simulink model "cSPACE_28335demo"  (R2017a)
settings: Solver=FixedStepDiscrete  StartTime=0.0  StopTime=inf  FixedStep=0.005  RelTol=1e-3  EnableMultiTasking=on
PostLoadFcn:
  | c2000demoscallback(1)
undefined symbols (not defined in the file or in its folder): Hardware_Interface, WM_DA0
libraries: idelinklib_common x16, simulink x4, c280xlib x2, c2833xlib x1
settings Model: ExtModeTrigDuration=8  Creator=The MathWorks Inc.  LastModifiedBy=307
settings DataIOCC: LimitDataPoints=on  SaveFormat=Array  SignalLoggingSaveFormat=ModelDataLogs  SaveOutput=off  SaveTime=off  SignalLoggingName=sigsOut
settings OptimizationCC: DefaultUnderspecifiedDataType=single  ExpressionDepthLimit=2147483647  InitFltsAndDblsToZero=on  LifeSpan=inf  MaxStackSize=512
settings DebuggingCC: UnderspecifiedInitializationDetection=Classic  MergeDetectMultiDrivingBlocksExec=none  CheckExecutionContextPreStartOutputMsg=on  CheckExecutionContextRuntimeOutputMsg=on  SignalResolutionControl=TryResolveAllWithWarning  MultiTaskDSMMsg=warning  MultiTaskCondExecSysMsg=none  SigSpecEnsureSampleTimeMsg=none  FcnCallInpInsideContextMsg=warning  StateNameClashWarn=warning  SFUnexpectedBacktrackingDiag=warning  SFNoUnconditionalDefaultTransitionDiag=warning  SFExecutionAtInitializationDiag=none
settings HardwareCC: ProdBitPerChar=16  ProdBitPerInt=16  ProdBitPerPointer=32  ProdBitPerSizeT=32  ProdBitPerPtrDiffT=32  ProdLargestAtomicInteger=Integer  ProdLargestAtomicFloat=None  ProdWordSize=16  ProdLongLongMode=on  ProdHWDeviceType=Texas Instruments->C2000  TargetBitPerChar=16  TargetBitPerInt=16  TargetLargestAtomicInteger=Integer  TargetIntDivRoundTo=Zero  TargetEndianess=LittleEndian  TargetWordSize=16  TargetHWDeviceType=Texas Instruments->C2000  ProdEqTarget=off
settings ModelReferenceCC: UpdateModelReferenceTargets=IfOutOfDate  PropagateSignalLabelsOutOfModel=off
settings SFSimCC: MATLABDynamicMemAlloc=off
settings RTWCC: SystemTargetFile=ert.tlc  HardwareBoard=TI Delfino F2833x  TLCOptions=-aInlineSetEventsForThisBaseRateFcn=TLC_FALSE -aSuppressMultiTaskScheduler=TLC_FALSE -aRateBasedStepFcn=1  TemplateMakefile=ert_default_tmf  Description=Embedded Coder  Toolchain=Texas Instruments Code Composer Studio v6 (C2000)
settings CodeAppCC: IgnoreCustomStorageClasses=off  CustomSymbolStrType=$N$R$M  InternalIdentifier=Classic
settings ERTTargetCC: CodeReplacementLibrary=TI C28x  MultiwordLength=2048  ParMdlRefBuildCompliant=off  SupportNonInlinedSFcns=on  CPPClassGenCompliant=off  ConvertIfToSwitch=off  SuppressUnreachableDefaultCases=off
settings ConfigComp: CovMetricSettings=dw  CovHtmlReporting=on  CovSaveCumulativeToWorkspaceVar=on  CovSaveSingleToWorkspaceVar=on  CovExternalEMLEnable=off  CovSFcnEnable=off

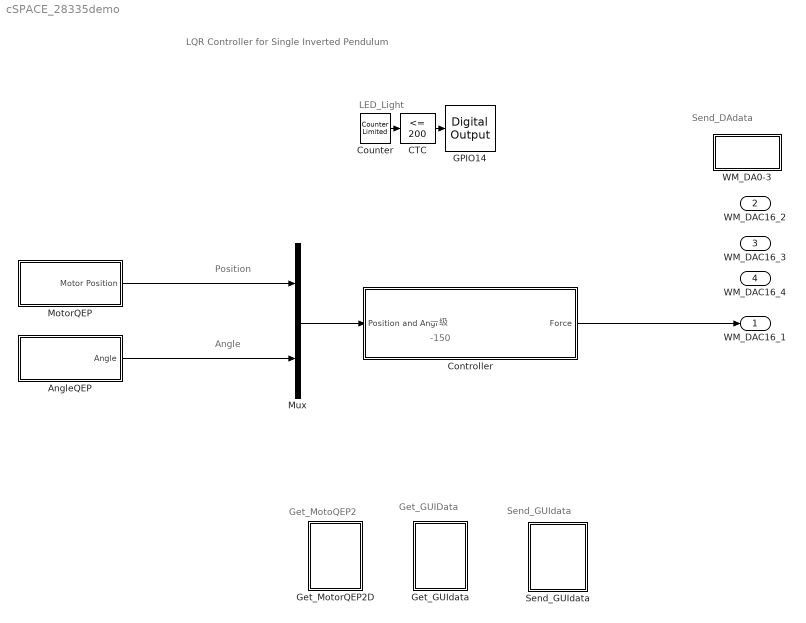
== system cSPACE_28335demo ==
  note: Send_GUIdata
  note: LED_Light
  note: Get_GUIData
  note: Send_DAdata
  note: Get_MotoQEP2
  note: LQR Controller for Single Inverted Pendulum
  note: -150
  note: 一级
  note: Position
  note: Angle
  " Controller" : Subsystem
  AngleQEP : Subsystem
  CTC : simulink/Logic and Bit Operations/Compare To Constant  relop=<=  const=200  OutDataTypeStr=boolean
  Counter : simulink/Sources/Counter Limited  uplimit=400  tsamp=-1
  GPIO14 : c2833xlib/Digital Output  GPIO_Number=GPIO8~GPIO15  GPIO_Bit0=off  GPIO_BIT0_Toggle=off  GPIO_Bit1=off  GPIO_BIT1_Toggle=off  GPIO_Bit2=off  GPIO_BIT2_Toggle=off  GPIO_Bit3=off  GPIO_BIT3_Toggle=off  GPIO_Bit4=off  GPIO_BIT4_Toggle=off  GPIO_Bit5=off  GPIO_BIT5_Toggle=off  GPIO_Bit6=on  GPIO_BIT6_Toggle=off  GPIO_Bit7=off  GPIO_BIT7_Toggle=off
      settings: SourceProductName=Embedded Coder Support Package for Texas Instruments C2000 Processors  SourceProductBaseCode=TIC2000
  Get_GUIdata : Subsystem
  Get_MotorQEP2D : Subsystem
  MotorQEP : Subsystem
  Mux : Mux  Inputs=2
  Send_GUIdata : Subsystem
  WM_DA0-3 : Subsystem  AncestorBlock=Hardware_Interface/WM_DA0-3  mask(The First channel of Encoder--WinnerMotor cSPACE){}
      mask help:
      | 33 MHz Clock Operation;
      | 32-Bit Binary Up/Down Counter
      mask Help: Please browse the web of winnermotor("http://www.winnermotor.com" ) for more information.
      mask Display: fprintf('WM\nDA0-3')
  WM_DAC16_1 : Outport
  WM_DAC16_2 : Outport  Port=2
  WM_DAC16_3 : Outport  Port=3
  WM_DAC16_4 : Outport  Port=4
  wires:
  Counter/1 -> CTC/1
  CTC/1 -> GPIO14/1
  " Controller"/1(Force) -> WM_DAC16_1/1
  MotorQEP/1(Motor Position) -> Mux/1
  Mux/1 -> " Controller"/1(Position and Angle)
  AngleQEP/1(Angle) -> Mux/2

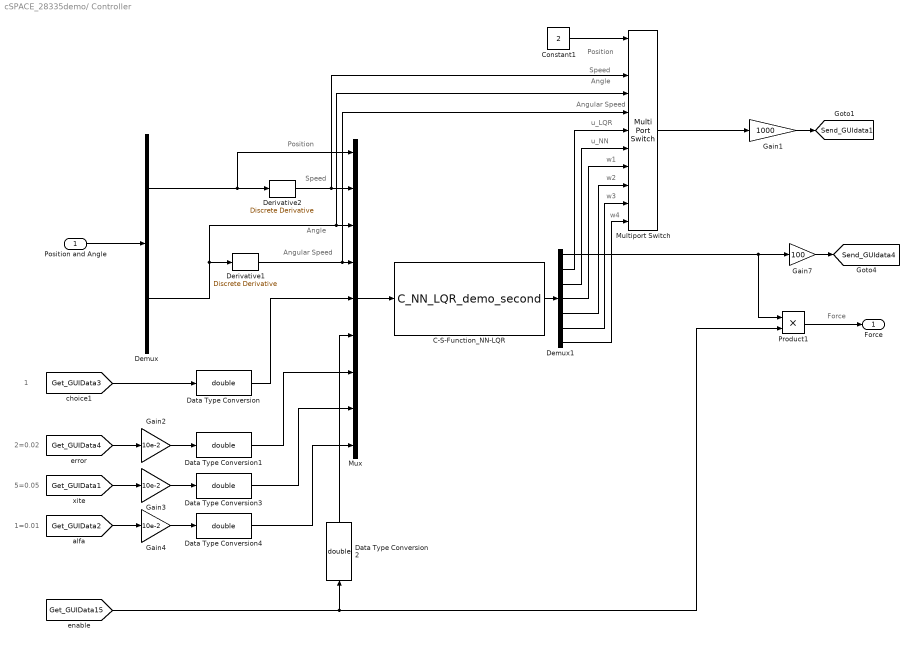
== system cSPACE_28335demo/ Controller ==
  note: Position
  note: Speed
  note: Angle
  note: Angular Speed
  note: Force
  note: Position
  note: Speed
  note: Angle
  note: Angular Speed
  note: u_LQR
  note: u_NN
  note: w1
  note: w2
  note: w3
  note: w4
  note: 5=0.05
  note: 1=0.01
  note: 2=0.02
  note: 1
  Position and Angle : Inport
  C-S-Function_NN-LQR : S-Function  FunctionName=C_NN_LQR_demo_second  SFunctionDeploymentMode=off  EnableBusSupport=off
  Constant1 : Constant  Value=2
  Data Type Conversion{,1..4} (5 alike) : DataTypeConversion  OutDataTypeStr=double
  Demux : Demux  Outputs=2
  Demux1 : Demux  Outputs=7
  Derivative1 : simulink/Discrete/Discrete Derivative  gainval=1.0  ICPrevScaledInput=0.0  InputProcessing=Inherited  OutMin=[]  OutMax=[]  OutDataType=sfix(16)  OutScaling=2^-10  DoSatur=off
  Derivative2 : simulink/Discrete/Discrete Derivative  gainval=1.0  ICPrevScaledInput=0.0  InputProcessing=Inherited  OutMin=[]  OutMax=[]  OutDataType=sfix(16)  OutScaling=2^-10  DoSatur=off
  Gain1 : Gain  Gain=1000
  Gain2 : Gain  Gain=10e-2  OutDataTypeStr=double
  Gain3 : Gain  Gain=10e-2  OutDataTypeStr=double
  Gain4 : Gain  Gain=10e-2  OutDataTypeStr=double
  Gain7 : Gain  Gain=100  OutDataTypeStr=double
  Multiport Switch : MultiPortSwitch  Inputs=10
  Mux : Mux  Inputs=9
  Product1 : Product
  Force : Outport
  tag scope: Send_GUIdata1=global, Send_GUIdata4=global
  wires:
  Product1/1 -> Force/1
  Derivative2/1 -> Mux/2, Multiport Switch/3
  Derivative1/1 -> Multiport Switch/5, Mux/4
  Demux/2 -> Mux/3, Multiport Switch/4, Derivative1/1
  Mux/1 -> C-S-Function_NN-LQR/1
  C-S-Function_NN-LQR/1 -> Demux1/1
  [Get_GUIData15] -> Data Type Conversion2/1, Product1/2
  Position and Angle/1 -> Demux/1
  Demux1/1 -> Product1/1, Gain7/1
  Demux1/2 -> Multiport Switch/6
  Demux1/3 -> Multiport Switch/7
  Demux1/4 -> Multiport Switch/8
  [Get_GUIData3] -> Data Type Conversion/1
  Data Type Conversion/1 -> Mux/5
  Demux1/5 -> Multiport Switch/9
  [Get_GUIData4] -> Gain2/1
  Data Type Conversion1/1 -> Mux/7
  Data Type Conversion2/1 -> Mux/6
  Gain2/1 -> Data Type Conversion1/1
  Gain3/1 -> Data Type Conversion3/1
  Data Type Conversion3/1 -> Mux/8
  [Get_GUIData1] -> Gain3/1
  [Get_GUIData2] -> Gain4/1
  Gain4/1 -> Data Type Conversion4/1
  Data Type Conversion4/1 -> Mux/9
  Demux1/6 -> Multiport Switch/10
  Demux1/7 -> Multiport Switch/11
  Constant1/1 -> Multiport Switch/1
  Multiport Switch/1 -> Gain1/1
  Gain7/1 -> [Send_GUIdata4]
  Gain1/1 -> [Send_GUIdata1]
  Demux/1 -> Mux/1, Derivative2/1

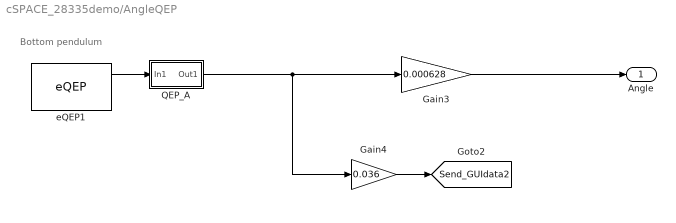
== system cSPACE_28335demo/AngleQEP ==
  note: Bottom pendulum
  Gain3 : Gain  Gain=0.000628
  Gain4 : Gain  Gain=0.036
  QEP_A : Subsystem
  eQEP1 : c280xlib/eQEP  useModule=eQEP1  pcInputmode=Quadrature-count  externalClockrate=2x resolution: Count the rising/falling edge  swapPolarityselection=Clockwise  qdfOutputport=off  qapPolarityselection=off  qbpPolarityselection=off  qipPolarityselection=off  qspPolarityselection=off  igatePolarityselection=off  sampleTime=-1  pcOutputport=on  pcMaximumvalue=65535  indexInitializationcheck=off  indexInitializationevent=Rising edge  strobeInitializationcheck=off  strobeInitializationevent=Rising edge  softwareInitializationcheck=on  softwareInitializationsource=Set to init value at start up  softwareInitializationmode=on  pcInitialvalue=27767  pcResetmode=Reset on the maximum position  ieloutputport=on  indexEventlatch=Falling edge  seloutputport=off  strobeEventlatch=Rising edge  pcefOutputport=off  enableEqepcapture=off  qctmrOutputport=off  qcprdOutputport=off  captureTimerprescaler=128  upEventprescaler=128  overflowErrorflag=off  directionErrorflag=off  captureTimerposition=On position counter read  unitTimerperiod=100000000  captureTimerlatch=off  capturePeriodlatch=off  positionCounterlatch=off  soenPolarityselection=off  spselPolarityselection=Index pin is used for sync output  compareValuesource=Specify via dialog  shadowMode=Load on QPOSCNT=0  compareValue=4294967295  syncOutputwidth=1  polaritySyncoutput=Active high  watchdogEnable=off  watchdogTimer=65535  outport1Datatype=uint8  outport2Datatype=uint16  outport3Datatype=uint16  outport4Datatype=auto  outport5Datatype=auto  outport6Datatype=auto  outport7Datatype=auto  outport8Datatype=auto  outport9Datatype=auto  outport10Datatype=auto  outport11Datatype=auto  outport12Datatype=auto  eqepinterrupt_pce=off  eqepinterrupt_qpe=off  eqepinterrupt_qdc=off  eqepinterrupt_wto=off  eqepinterrupt_pcu=off  eqepinterrupt_pco=off  eqepinterrupt_pcr=off  eqepinterrupt_pcm=off  eqepinterrupt_sel=off  eqepinterrupt_iel=off  eqepinterrupt_uto=off  pheOutputport=off  watchdogOutputport=off  outport13Datatype=auto  outport14Datatype=auto
      settings: SourceProductName=Embedded Coder Support Package for Texas Instruments C2000 Processors  SourceProductBaseCode=TIC2000
  Angle : Outport
  tag scope: Send_GUIdata2=global
  wires:
  QEP_A/1(Out1) -> Gain3/1, Gain4/1
  eQEP1/1 -> QEP_A/1(In1)
  Gain3/1 -> Angle/1
  Gain4/1 -> [Send_GUIdata2]

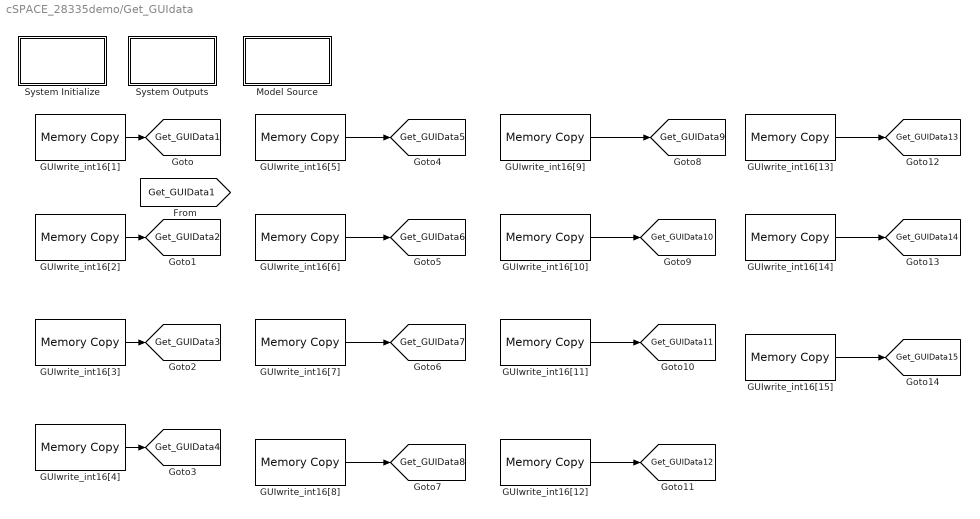
== system cSPACE_28335demo/Get_GUIdata ==
  GUIwrite_int16[10] : idelinklib_common/Memory Copy  copyFrom=Specified source code symbol  copyFromAddressSource=Specify via dialog  copyFromAddress=hex2dec('00001000')  copyFromSrcCode=&GUIwrite_int16[10]  dataTypeFrom=uint16  dataDimensionFrom=1  useOffsetFrom=off  offsetFromSrc=Specify via dialog  offsetFrom=1  strideFrom=1  copyTo=Output port  copyToAddressSource=Specify via dialog  copyToAddress=hex2dec('00002000')  copyToSrcCode=myVariableDst  dataTypeTo=int16  useOffsetTo=off  offsetToSrc=Specify via dialog  offsetTo=1  strideTo=1  sampleTime=-1  useInitValue=off  initValueSrc=Specify constant value  initValue=1  initValueSrcCode=myInitValueVariable  useAsMask=off  maskOperator=bitwise AND  useTermValue=off  termValue=1  isRealtimeEnabled=off  emitCCBeforeWrite=on  CCBeforeWrite=/* Custom Code Before Write*/  emitCCAfterWrite=on  CCAfterWrite=/* Custom Code After Write*/  useDMACopy=off  enableBlockingMode=off
  GUIwrite_int16[11] : idelinklib_common/Memory Copy  copyFrom=Specified source code symbol  copyFromAddressSource=Specify via dialog  copyFromAddress=hex2dec('00001000')  copyFromSrcCode=&GUIwrite_int16[11]  dataTypeFrom=uint16  dataDimensionFrom=1  useOffsetFrom=off  offsetFromSrc=Specify via dialog  offsetFrom=1  strideFrom=1  copyTo=Output port  copyToAddressSource=Specify via dialog  copyToAddress=hex2dec('00002000')  copyToSrcCode=myVariableDst  dataTypeTo=int16  useOffsetTo=off  offsetToSrc=Specify via dialog  offsetTo=1  strideTo=1  sampleTime=-1  useInitValue=off  initValueSrc=Specify constant value  initValue=1  initValueSrcCode=myInitValueVariable  useAsMask=off  maskOperator=bitwise AND  useTermValue=off  termValue=1  isRealtimeEnabled=off  emitCCBeforeWrite=on  CCBeforeWrite=/* Custom Code Before Write*/  emitCCAfterWrite=on  CCAfterWrite=/* Custom Code After Write*/  useDMACopy=off  enableBlockingMode=off
  GUIwrite_int16[12] : idelinklib_common/Memory Copy  copyFrom=Specified source code symbol  copyFromAddressSource=Specify via dialog  copyFromAddress=hex2dec('00001000')  copyFromSrcCode=&GUIwrite_int16[12]  dataTypeFrom=uint16  dataDimensionFrom=1  useOffsetFrom=off  offsetFromSrc=Specify via dialog  offsetFrom=1  strideFrom=1  copyTo=Output port  copyToAddressSource=Specify via dialog  copyToAddress=hex2dec('00002000')  copyToSrcCode=myVariableDst  dataTypeTo=int16  useOffsetTo=off  offsetToSrc=Specify via dialog  offsetTo=1  strideTo=1  sampleTime=-1  useInitValue=off  initValueSrc=Specify constant value  initValue=1  initValueSrcCode=myInitValueVariable  useAsMask=off  maskOperator=bitwise AND  useTermValue=off  termValue=1  isRealtimeEnabled=off  emitCCBeforeWrite=on  CCBeforeWrite=/* Custom Code Before Write*/  emitCCAfterWrite=on  CCAfterWrite=/* Custom Code After Write*/  useDMACopy=off  enableBlockingMode=off
  GUIwrite_int16[13] : idelinklib_common/Memory Copy  copyFrom=Specified source code symbol  copyFromAddressSource=Specify via dialog  copyFromAddress=hex2dec('00001000')  copyFromSrcCode=&GUIwrite_int16[13]  dataTypeFrom=uint16  dataDimensionFrom=1  useOffsetFrom=off  offsetFromSrc=Specify via dialog  offsetFrom=1  strideFrom=1  copyTo=Output port  copyToAddressSource=Specify via dialog  copyToAddress=hex2dec('00002000')  copyToSrcCode=myVariableDst  dataTypeTo=int16  useOffsetTo=off  offsetToSrc=Specify via dialog  offsetTo=1  strideTo=1  sampleTime=-1  useInitValue=off  initValueSrc=Specify constant value  initValue=1  initValueSrcCode=myInitValueVariable  useAsMask=off  maskOperator=bitwise AND  useTermValue=off  termValue=1  isRealtimeEnabled=off  emitCCBeforeWrite=on  CCBeforeWrite=/* Custom Code Before Write*/  emitCCAfterWrite=on  CCAfterWrite=/* Custom Code After Write*/  useDMACopy=off  enableBlockingMode=off
  GUIwrite_int16[14] : idelinklib_common/Memory Copy  copyFrom=Specified source code symbol  copyFromAddressSource=Specify via dialog  copyFromAddress=hex2dec('00001000')  copyFromSrcCode=&GUIwrite_int16[14]  dataTypeFrom=uint16  dataDimensionFrom=1  useOffsetFrom=off  offsetFromSrc=Specify via dialog  offsetFrom=1  strideFrom=1  copyTo=Output port  copyToAddressSource=Specify via dialog  copyToAddress=hex2dec('00002000')  copyToSrcCode=myVariableDst  dataTypeTo=int16  useOffsetTo=off  offsetToSrc=Specify via dialog  offsetTo=1  strideTo=1  sampleTime=-1  useInitValue=off  initValueSrc=Specify constant value  initValue=1  initValueSrcCode=myInitValueVariable  useAsMask=off  maskOperator=bitwise AND  useTermValue=off  termValue=1  isRealtimeEnabled=off  emitCCBeforeWrite=on  CCBeforeWrite=/* Custom Code Before Write*/  emitCCAfterWrite=on  CCAfterWrite=/* Custom Code After Write*/  useDMACopy=off  enableBlockingMode=off
  GUIwrite_int16[15] : idelinklib_common/Memory Copy  copyFrom=Specified source code symbol  copyFromAddressSource=Specify via dialog  copyFromAddress=hex2dec('00001000')  copyFromSrcCode=&GUIwrite_int16[15]  dataTypeFrom=uint16  dataDimensionFrom=1  useOffsetFrom=off  offsetFromSrc=Specify via dialog  offsetFrom=1  strideFrom=1  copyTo=Output port  copyToAddressSource=Specify via dialog  copyToAddress=hex2dec('00002000')  copyToSrcCode=myVariableDst  dataTypeTo=int16  useOffsetTo=off  offsetToSrc=Specify via dialog  offsetTo=1  strideTo=1  sampleTime=-1  useInitValue=off  initValueSrc=Specify constant value  initValue=1  initValueSrcCode=myInitValueVariable  useAsMask=off  maskOperator=bitwise AND  useTermValue=off  termValue=1  isRealtimeEnabled=off  emitCCBeforeWrite=on  CCBeforeWrite=/* Custom Code Before Write*/  emitCCAfterWrite=on  CCAfterWrite=/* Custom Code After Write*/  useDMACopy=off  enableBlockingMode=off
  GUIwrite_int16[1] : idelinklib_common/Memory Copy  copyFrom=Specified source code symbol  copyFromAddressSource=Specify via dialog  copyFromAddress=hex2dec('00001000')  copyFromSrcCode=&GUIwrite_int16[1]  dataTypeFrom=uint16  dataDimensionFrom=1  useOffsetFrom=off  offsetFromSrc=Specify via dialog  offsetFrom=1  strideFrom=1  copyTo=Output port  copyToAddressSource=Specify via dialog  copyToAddress=hex2dec('00002000')  copyToSrcCode=myVariableDst  dataTypeTo=int16  useOffsetTo=off  offsetToSrc=Specify via dialog  offsetTo=1  strideTo=1  sampleTime=-1  useInitValue=off  initValueSrc=Specify constant value  initValue=1  initValueSrcCode=myInitValueVariable  useAsMask=off  maskOperator=bitwise AND  useTermValue=off  termValue=1  isRealtimeEnabled=off  emitCCBeforeWrite=on  CCBeforeWrite=/* Custom Code Before Write*/  emitCCAfterWrite=on  CCAfterWrite=/* Custom Code After Write*/  useDMACopy=off  enableBlockingMode=off
  GUIwrite_int16[2] : idelinklib_common/Memory Copy  copyFrom=Specified source code symbol  copyFromAddressSource=Specify via dialog  copyFromAddress=hex2dec('00001000')  copyFromSrcCode=&GUIwrite_int16[2]  dataTypeFrom=uint16  dataDimensionFrom=1  useOffsetFrom=off  offsetFromSrc=Specify via dialog  offsetFrom=1  strideFrom=1  copyTo=Output port  copyToAddressSource=Specify via dialog  copyToAddress=hex2dec('00002000')  copyToSrcCode=myVariableDst  dataTypeTo=int16  useOffsetTo=off  offsetToSrc=Specify via dialog  offsetTo=1  strideTo=1  sampleTime=-1  useInitValue=off  initValueSrc=Specify constant value  initValue=1  initValueSrcCode=myInitValueVariable  useAsMask=off  maskOperator=bitwise AND  useTermValue=off  termValue=1  isRealtimeEnabled=off  emitCCBeforeWrite=on  CCBeforeWrite=/* Custom Code Before Write*/  emitCCAfterWrite=on  CCAfterWrite=/* Custom Code After Write*/  useDMACopy=off  enableBlockingMode=off
  GUIwrite_int16[3] : idelinklib_common/Memory Copy  copyFrom=Specified source code symbol  copyFromAddressSource=Specify via dialog  copyFromAddress=hex2dec('00001000')  copyFromSrcCode=&GUIwrite_int16[3]  dataTypeFrom=uint16  dataDimensionFrom=1  useOffsetFrom=off  offsetFromSrc=Specify via dialog  offsetFrom=1  strideFrom=1  copyTo=Output port  copyToAddressSource=Specify via dialog  copyToAddress=hex2dec('00002000')  copyToSrcCode=myVariableDst  dataTypeTo=int16  useOffsetTo=off  offsetToSrc=Specify via dialog  offsetTo=1  strideTo=1  sampleTime=-1  useInitValue=off  initValueSrc=Specify constant value  initValue=1  initValueSrcCode=myInitValueVariable  useAsMask=off  maskOperator=bitwise AND  useTermValue=off  termValue=1  isRealtimeEnabled=off  emitCCBeforeWrite=on  CCBeforeWrite=/* Custom Code Before Write*/  emitCCAfterWrite=on  CCAfterWrite=/* Custom Code After Write*/  useDMACopy=off  enableBlockingMode=off
  GUIwrite_int16[4] : idelinklib_common/Memory Copy  copyFrom=Specified source code symbol  copyFromAddressSource=Specify via dialog  copyFromAddress=hex2dec('00001000')  copyFromSrcCode=&GUIwrite_int16[4]  dataTypeFrom=uint16  dataDimensionFrom=1  useOffsetFrom=off  offsetFromSrc=Specify via dialog  offsetFrom=1  strideFrom=1  copyTo=Output port  copyToAddressSource=Specify via dialog  copyToAddress=hex2dec('00002000')  copyToSrcCode=myVariableDst  dataTypeTo=int16  useOffsetTo=off  offsetToSrc=Specify via dialog  offsetTo=1  strideTo=1  sampleTime=-1  useInitValue=off  initValueSrc=Specify constant value  initValue=1  initValueSrcCode=myInitValueVariable  useAsMask=off  maskOperator=bitwise AND  useTermValue=off  termValue=1  isRealtimeEnabled=off  emitCCBeforeWrite=on  CCBeforeWrite=/* Custom Code Before Write*/  emitCCAfterWrite=on  CCAfterWrite=/* Custom Code After Write*/  useDMACopy=off  enableBlockingMode=off
  GUIwrite_int16[5] : idelinklib_common/Memory Copy  copyFrom=Specified source code symbol  copyFromAddressSource=Specify via dialog  copyFromAddress=hex2dec('00001000')  copyFromSrcCode=&GUIwrite_int16[5]  dataTypeFrom=uint16  dataDimensionFrom=1  useOffsetFrom=off  offsetFromSrc=Specify via dialog  offsetFrom=1  strideFrom=1  copyTo=Output port  copyToAddressSource=Specify via dialog  copyToAddress=hex2dec('00002000')  copyToSrcCode=myVariableDst  dataTypeTo=int16  useOffsetTo=off  offsetToSrc=Specify via dialog  offsetTo=1  strideTo=1  sampleTime=-1  useInitValue=off  initValueSrc=Specify constant value  initValue=1  initValueSrcCode=myInitValueVariable  useAsMask=off  maskOperator=bitwise AND  useTermValue=off  termValue=1  isRealtimeEnabled=off  emitCCBeforeWrite=on  CCBeforeWrite=/* Custom Code Before Write*/  emitCCAfterWrite=on  CCAfterWrite=/* Custom Code After Write*/  useDMACopy=off  enableBlockingMode=off
  GUIwrite_int16[6] : idelinklib_common/Memory Copy  copyFrom=Specified source code symbol  copyFromAddressSource=Specify via dialog  copyFromAddress=hex2dec('00001000')  copyFromSrcCode=&GUIwrite_int16[6]  dataTypeFrom=uint16  dataDimensionFrom=1  useOffsetFrom=off  offsetFromSrc=Specify via dialog  offsetFrom=1  strideFrom=1  copyTo=Output port  copyToAddressSource=Specify via dialog  copyToAddress=hex2dec('00002000')  copyToSrcCode=myVariableDst  dataTypeTo=int16  useOffsetTo=off  offsetToSrc=Specify via dialog  offsetTo=1  strideTo=1  sampleTime=-1  useInitValue=off  initValueSrc=Specify constant value  initValue=1  initValueSrcCode=myInitValueVariable  useAsMask=off  maskOperator=bitwise AND  useTermValue=off  termValue=1  isRealtimeEnabled=off  emitCCBeforeWrite=on  CCBeforeWrite=/* Custom Code Before Write*/  emitCCAfterWrite=on  CCAfterWrite=/* Custom Code After Write*/  useDMACopy=off  enableBlockingMode=off
  GUIwrite_int16[7] : idelinklib_common/Memory Copy  copyFrom=Specified source code symbol  copyFromAddressSource=Specify via dialog  copyFromAddress=hex2dec('00001000')  copyFromSrcCode=&GUIwrite_int16[7]  dataTypeFrom=uint16  dataDimensionFrom=1  useOffsetFrom=off  offsetFromSrc=Specify via dialog  offsetFrom=1  strideFrom=1  copyTo=Output port  copyToAddressSource=Specify via dialog  copyToAddress=hex2dec('00002000')  copyToSrcCode=myVariableDst  dataTypeTo=int16  useOffsetTo=off  offsetToSrc=Specify via dialog  offsetTo=1  strideTo=1  sampleTime=-1  useInitValue=off  initValueSrc=Specify constant value  initValue=1  initValueSrcCode=myInitValueVariable  useAsMask=off  maskOperator=bitwise AND  useTermValue=off  termValue=1  isRealtimeEnabled=off  emitCCBeforeWrite=on  CCBeforeWrite=/* Custom Code Before Write*/  emitCCAfterWrite=on  CCAfterWrite=/* Custom Code After Write*/  useDMACopy=off  enableBlockingMode=off
  GUIwrite_int16[8] : idelinklib_common/Memory Copy  copyFrom=Specified source code symbol  copyFromAddressSource=Specify via dialog  copyFromAddress=hex2dec('00001000')  copyFromSrcCode=&GUIwrite_int16[8]  dataTypeFrom=uint16  dataDimensionFrom=1  useOffsetFrom=off  offsetFromSrc=Specify via dialog  offsetFrom=1  strideFrom=1  copyTo=Output port  copyToAddressSource=Specify via dialog  copyToAddress=hex2dec('00002000')  copyToSrcCode=myVariableDst  dataTypeTo=int16  useOffsetTo=off  offsetToSrc=Specify via dialog  offsetTo=1  strideTo=1  sampleTime=-1  useInitValue=off  initValueSrc=Specify constant value  initValue=1  initValueSrcCode=myInitValueVariable  useAsMask=off  maskOperator=bitwise AND  useTermValue=off  termValue=1  isRealtimeEnabled=off  emitCCBeforeWrite=on  CCBeforeWrite=/* Custom Code Before Write*/  emitCCAfterWrite=on  CCAfterWrite=/* Custom Code After Write*/  useDMACopy=off  enableBlockingMode=off
  GUIwrite_int16[9] : idelinklib_common/Memory Copy  copyFrom=Specified source code symbol  copyFromAddressSource=Specify via dialog  copyFromAddress=hex2dec('00001000')  copyFromSrcCode=&GUIwrite_int16[9]  dataTypeFrom=uint16  dataDimensionFrom=1  useOffsetFrom=off  offsetFromSrc=Specify via dialog  offsetFrom=1  strideFrom=1  copyTo=Output port  copyToAddressSource=Specify via dialog  copyToAddress=hex2dec('00002000')  copyToSrcCode=myVariableDst  dataTypeTo=int16  useOffsetTo=off  offsetToSrc=Specify via dialog  offsetTo=1  strideTo=1  sampleTime=-1  useInitValue=off  initValueSrc=Specify constant value  initValue=1  initValueSrcCode=myInitValueVariable  useAsMask=off  maskOperator=bitwise AND  useTermValue=off  termValue=1  isRealtimeEnabled=off  emitCCBeforeWrite=on  CCBeforeWrite=/* Custom Code Before Write*/  emitCCAfterWrite=on  CCAfterWrite=/* Custom Code After Write*/  useDMACopy=off  enableBlockingMode=off
  Model Source : Subsystem  mask(Model Source){ShowInLibBrowser=0}
      mask prompts: ShowInLibBrowser "Mask Parameter 1:"
      mask help: Add code to the model .c file
      settings: CopyFcn=cccopyfcn(gcb)  OpenFcn=ccopenfcn('Model Source')
      mask Help: eval('feval(''rtwprivate'',''rtwhelpview'',''rtw_model_source_block'')');
      mask Display: disp('Model\nSource');
  System Initialize : Subsystem  mask(System Initialize){ShowInLibBrowser=0}
      mask prompts: ShowInLibBrowser "Mask Parameter 1:"
      mask help: Add code to a systems Initialize function
      settings: CopyFcn=cccopyfcn(gcb)  OpenFcn=ccopenfcn('System Initialize Function')
      mask Help: eval('feval(''rtwprivate'',''rtwhelpview'',''rtw_sys_initialize_block'')');
      mask Display: disp('System\nInitialize');
  System Outputs : Subsystem  mask(System Outputs){ShowInLibBrowser=0}
      mask prompts: ShowInLibBrowser "Mask Parameter 1:"
      mask help: Add code to a systems Outputs function
      settings: CopyFcn=cccopyfcn(gcb)  OpenFcn=ccopenfcn('System Outputs Function')
      mask Help: eval('feval(''rtwprivate'',''rtwhelpview'',''rtw_sys_outputs_block'')');
      mask Display: disp('System\nOutputs');
  tag scope: Get_GUIData10=global, Get_GUIData11=global, Get_GUIData12=global, Get_GUIData13=global, Get_GUIData14=global, Get_GUIData15=global, Get_GUIData1=global, Get_GUIData2=global, Get_GUIData3=global, Get_GUIData4=global, Get_GUIData5=global, Get_GUIData6=global, Get_GUIData7=global, Get_GUIData8=global, Get_GUIData9=global
  wires:
  GUIwrite_int16[1]/1 -> [Get_GUIData1]
  GUIwrite_int16[2]/1 -> [Get_GUIData2]
  GUIwrite_int16[3]/1 -> [Get_GUIData3]
  GUIwrite_int16[4]/1 -> [Get_GUIData4]
  GUIwrite_int16[5]/1 -> [Get_GUIData5]
  GUIwrite_int16[6]/1 -> [Get_GUIData6]
  GUIwrite_int16[7]/1 -> [Get_GUIData7]
  GUIwrite_int16[8]/1 -> [Get_GUIData8]
  GUIwrite_int16[9]/1 -> [Get_GUIData9]
  GUIwrite_int16[10]/1 -> [Get_GUIData10]
  GUIwrite_int16[11]/1 -> [Get_GUIData11]
  GUIwrite_int16[12]/1 -> [Get_GUIData12]
  GUIwrite_int16[13]/1 -> [Get_GUIData13]
  GUIwrite_int16[14]/1 -> [Get_GUIData14]
  GUIwrite_int16[15]/1 -> [Get_GUIData15]

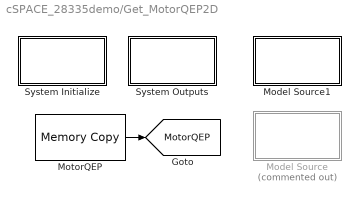
== system cSPACE_28335demo/Get_MotorQEP2D ==
  Model Source : Subsystem  Commented=on  mask(Model Source){ShowInLibBrowser=0}
      mask prompts: ShowInLibBrowser "Mask Parameter 1:"
      mask help: Add code to the model .c file
      settings: CopyFcn=cccopyfcn(gcb)  OpenFcn=ccopenfcn('Model Source')
      mask Help: eval('feval(''rtwprivate'',''rtwhelpview'',''rtw_model_source_block'')');
      mask Display: disp('Model\nSource');
  Model Source1 : Subsystem  mask(Model Source){ShowInLibBrowser=0}
      mask prompts: ShowInLibBrowser "Mask Parameter 1:"
      mask help: Add code to the model .c file
      settings: CopyFcn=cccopyfcn(gcb)  OpenFcn=ccopenfcn('Model Source')
      mask Help: eval('feval(''rtwprivate'',''rtwhelpview'',''rtw_model_source_block'')');
      mask Display: disp('Model\nSource');
  MotorQEP : idelinklib_common/Memory Copy  copyFrom=Specified source code symbol  copyFromAddressSource=Specify via dialog  copyFromAddress=hex2dec('00001000')  copyFromSrcCode=&eCANReceive_dataL  dataTypeFrom=uint32  dataDimensionFrom=1  useOffsetFrom=off  offsetFromSrc=Specify via dialog  offsetFrom=1  strideFrom=1  copyTo=Output port  copyToAddressSource=Specify via dialog  copyToAddress=hex2dec('00002000')  copyToSrcCode=myVariableDst  dataTypeTo=uint32  useOffsetTo=off  offsetToSrc=Specify via dialog  offsetTo=1  strideTo=1  sampleTime=-1  useInitValue=off  initValueSrc=Specify constant value  initValue=1  initValueSrcCode=myInitValueVariable  useAsMask=off  maskOperator=bitwise AND  useTermValue=off  termValue=1  isRealtimeEnabled=off  emitCCBeforeWrite=on  CCBeforeWrite=/* Custom Code Before Write*/  emitCCAfterWrite=on  CCAfterWrite=/* Custom Code After Write*/  useDMACopy=off  enableBlockingMode=off
  System Initialize : Subsystem  mask(System Initialize){ShowInLibBrowser=0}
      mask prompts: ShowInLibBrowser "Mask Parameter 1:"
      mask help: Add code to a systems Initialize function
      settings: CopyFcn=cccopyfcn(gcb)  OpenFcn=ccopenfcn('System Initialize Function')
      mask Help: eval('feval(''rtwprivate'',''rtwhelpview'',''rtw_sys_initialize_block'')');
      mask Display: disp('System\nInitialize');
  System Outputs : Subsystem  mask(System Outputs){ShowInLibBrowser=0}
      mask prompts: ShowInLibBrowser "Mask Parameter 1:"
      mask help: Add code to a systems Outputs function
      settings: CopyFcn=cccopyfcn(gcb)  OpenFcn=ccopenfcn('System Outputs Function')
      mask Help: eval('feval(''rtwprivate'',''rtwhelpview'',''rtw_sys_outputs_block'')');
      mask Display: disp('System\nOutputs');
  tag scope: MotorQEP=global
  wires:
  MotorQEP/1 -> [MotorQEP]

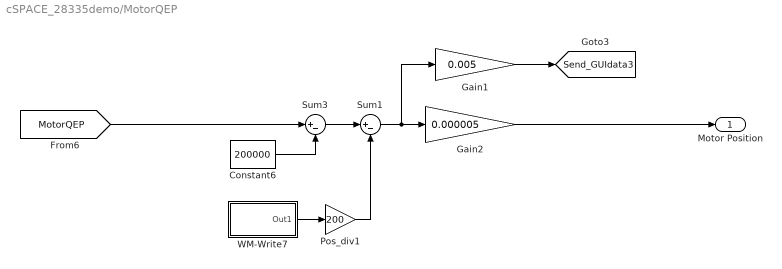
== system cSPACE_28335demo/MotorQEP ==
  Constant6 : Constant  Value=200000  OutDataTypeStr=double
  Gain1 : Gain  Gain=0.005
  Gain2 : Gain  Gain=0.000005
  Pos_div1 : Gain  Gain=200
  Sum1 : Sum  Inputs=|+-
  Sum3 : Sum  Inputs=|+-
  WM-Write7 : Subsystem
  Motor Position : Outport
  tag scope: Send_GUIdata3=global
  wires:
  Constant6/1 -> Sum3/2
  Pos_div1/1 -> Sum1/2
  Sum3/1 -> Sum1/1
  Sum1/1 -> Gain2/1, Gain1/1
  [MotorQEP] -> Sum3/1
  WM-Write7/1(Out1) -> Pos_div1/1
  Gain2/1 -> Motor Position/1
  Gain1/1 -> [Send_GUIdata3]

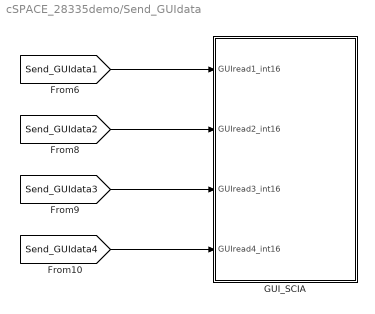
== system cSPACE_28335demo/Send_GUIdata ==
  GUI_SCIA : Subsystem
  wires:
  [Send_GUIdata1] -> GUI_SCIA/1(GUIread1_int16)
  [Send_GUIdata2] -> GUI_SCIA/2(GUIread2_int16)
  [Send_GUIdata3] -> GUI_SCIA/3(GUIread3_int16)
  [Send_GUIdata4] -> GUI_SCIA/4(GUIread4_int16)

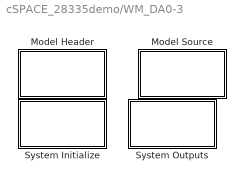
== system cSPACE_28335demo/WM_DA0-3 ==
  Model Header : Subsystem  mask(Model Header){ShowInLibBrowser=0}
      mask prompts: ShowInLibBrowser "Mask Parameter 1:"
      mask help: Add code to the model .h file
      settings: CopyFcn=cccopyfcn(gcb)  OpenFcn=ccopenfcn('Model Header')
      mask Help: eval('feval(''rtwprivate'',''rtwhelpview'',''rtw_model_header_block'')');
      mask Display: disp('Model\nHeader');
  Model Source : Subsystem  mask(Model Source){ShowInLibBrowser=0}
      mask prompts: ShowInLibBrowser "Mask Parameter 1:"
      mask help: Add code to the model .c file
      settings: CopyFcn=cccopyfcn(gcb)  OpenFcn=ccopenfcn('Model Source')
      mask Help: helpview([docroot '/toolbox/rtw/helptargets.map'], 'rtw_model_source_block');
      mask Display: disp('Model\nSource');
  System Initialize : Subsystem  mask(System Initialize){ShowInLibBrowser=0}
      mask prompts: ShowInLibBrowser "Mask Parameter 1:"
      mask help: Add code to a systems Initialize function
      settings: CopyFcn=cccopyfcn(gcb)  OpenFcn=ccopenfcn('System Initialize Function')
      mask Help: helpview([docroot '/toolbox/rtw/helptargets.map'], 'rtw_sys_initialize_block');
      mask Display: disp('System\nInitialize');
  System Outputs : Subsystem  mask(System Outputs){ShowInLibBrowser=0}
      mask prompts: ShowInLibBrowser "Mask Parameter 1:"
      mask help: Add code to a systems Outputs function
      settings: CopyFcn=cccopyfcn(gcb)  OpenFcn=ccopenfcn('System Outputs Function')
      mask Help: helpview([docroot '/toolbox/rtw/helptargets.map'], 'rtw_sys_outputs_block');
      mask Display: disp('System\nOutputs');

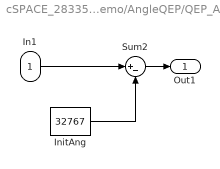
== system cSPACE_28335demo/AngleQEP/QEP_A ==
  In1 : Inport
  InitAng : Constant  Value=32767
  Sum2 : Sum  Inputs=|+-
  Out1 : Outport
  wires:
  Sum2/1 -> Out1/1
  InitAng/1 -> Sum2/2
  In1/1 -> Sum2/1

== system cSPACE_28335demo/Get_GUIdata/Model Source ==

== system cSPACE_28335demo/Get_GUIdata/System Initialize ==

== system cSPACE_28335demo/Get_GUIdata/System Outputs ==

== system cSPACE_28335demo/Get_MotorQEP2D/Model Source ==

== system cSPACE_28335demo/Get_MotorQEP2D/Model Source1 ==

== system cSPACE_28335demo/Get_MotorQEP2D/System Initialize ==

== system cSPACE_28335demo/Get_MotorQEP2D/System Outputs ==

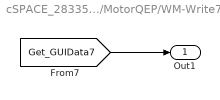
== system cSPACE_28335demo/MotorQEP/WM-Write7 ==
  Out1 : Outport
  wires:
  [Get_GUIData7] -> Out1/1

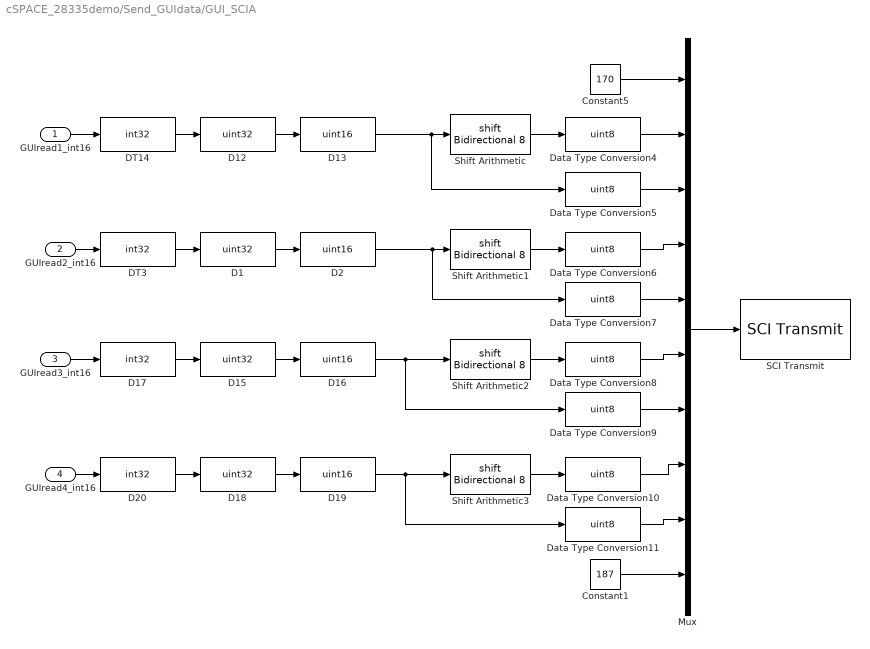
== system cSPACE_28335demo/Send_GUIdata/GUI_SCIA ==
  GUIread1_int16 : Inport
  GUIread2_int16 : Inport  Port=2
  GUIread3_int16 : Inport  Port=3
  GUIread4_int16 : Inport  Port=4
  Constant1 : Constant  Value=187  OutDataTypeStr=uint8
  Constant5 : Constant  Value=170  OutDataTypeStr=uint8
  D{1,12,15,18} (4 alike) : DataTypeConversion  OutDataTypeStr=uint32
  D{2,13,16,19} (4 alike) : DataTypeConversion  OutDataTypeStr=uint16
  D17 : DataTypeConversion  OutDataTypeStr=int32
  D20 : DataTypeConversion  OutDataTypeStr=int32
  DT14 : DataTypeConversion  OutDataTypeStr=int32
  DT3 : DataTypeConversion  OutDataTypeStr=int32
  Data Type Conversion{4..11} (8 alike) : DataTypeConversion  OutDataTypeStr=uint8
  Mux : Mux  Inputs=10
  SCI Transmit : c280xlib/SCI Transmit  sciModule=A  dataHead=''  dataTail=''  postInterrupt=on  numFifo=16
      settings: SourceProductName=Embedded Coder Support Package for Texas Instruments C2000 Processors
  Shift Arithmetic{,1..3} (4 alike) : ArithShift  BitShiftNumber=8
  wires:
  D13/1 -> Data Type Conversion5/1, Shift Arithmetic/1
  Data Type Conversion10/1 -> Mux/8
  Data Type Conversion6/1 -> Mux/4
  Constant1/1 -> Mux/10
  Data Type Conversion11/1 -> Mux/9
  Shift Arithmetic2/1 -> Data Type Conversion8/1
  D1/1 -> D2/1
  D2/1 -> Data Type Conversion7/1, Shift Arithmetic1/1
  D16/1 -> Data Type Conversion9/1, Shift Arithmetic2/1
  Shift Arithmetic1/1 -> Data Type Conversion6/1
  Shift Arithmetic/1 -> Data Type Conversion4/1
  Data Type Conversion4/1 -> Mux/2
  DT3/1 -> D1/1
  Data Type Conversion8/1 -> Mux/6
  Data Type Conversion5/1 -> Mux/3
  GUIread2_int16/1 -> DT3/1
  Constant5/1 -> Mux/1
  Data Type Conversion7/1 -> Mux/5
  Shift Arithmetic3/1 -> Data Type Conversion10/1
  D19/1 -> Data Type Conversion11/1, Shift Arithmetic3/1
  Mux/1 -> SCI Transmit/1
  Data Type Conversion9/1 -> Mux/7
  DT14/1 -> D12/1
  GUIread1_int16/1 -> DT14/1
  D12/1 -> D13/1
  D17/1 -> D15/1
  GUIread3_int16/1 -> D17/1
  D15/1 -> D16/1
  D20/1 -> D18/1
  GUIread4_int16/1 -> D20/1
  D18/1 -> D19/1

== system cSPACE_28335demo/WM_DA0-3/Model Header ==

== system cSPACE_28335demo/WM_DA0-3/Model Source ==

== system cSPACE_28335demo/WM_DA0-3/System Initialize ==

== system cSPACE_28335demo/WM_DA0-3/System Outputs ==
